simulink model "Ejemplo_01_simulink"  (R2018a)
settings: Solver=VariableStepAuto  StartTime=0.0  StopTime=10.0  RelTol=1e-3
settings Model: Creator=LENOVO  LastModifiedBy=LENOVO

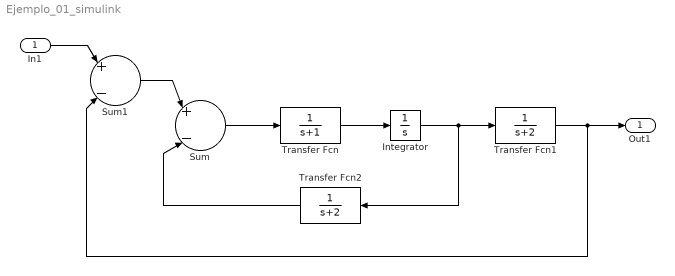
== system Ejemplo_01_simulink ==
  In1 : Inport
  Integrator : Integrator
  Sum : Sum  Inputs=|+|-|
  Sum1 : Sum  Inputs=|+|-|
  Transfer Fcn : TransferFcn  Denominator=[1 1]
  Transfer Fcn1 : TransferFcn  Denominator=[1 2]
  Transfer Fcn2 : TransferFcn  Denominator=[1 2]
  Out1 : Outport
  wires:
  Sum/1 -> Transfer Fcn/1
  Transfer Fcn/1 -> Integrator/1
  Integrator/1 -> Transfer Fcn2/1, Transfer Fcn1/1
  Sum1/1 -> Sum/1
  Transfer Fcn2/1 -> Sum/2
  In1/1 -> Sum1/1
  Transfer Fcn1/1 -> Sum1/2, Out1/1
